simulink model "RC_Model"  (R2023b)
settings: Solver=VariableStepAuto  StartTime=0.0  StopTime=10.0  MaxStep=1e-3  RelTol=1e-3
values from neighbouring files (symbols this model uses):
  C = 1*10^-6    (= 1e-06)    [Script_Rc_model.m]
  R = 1    [Script_Rc_model.m]
settings Model: Creator=gaafa  LastModifiedBy=gaafa

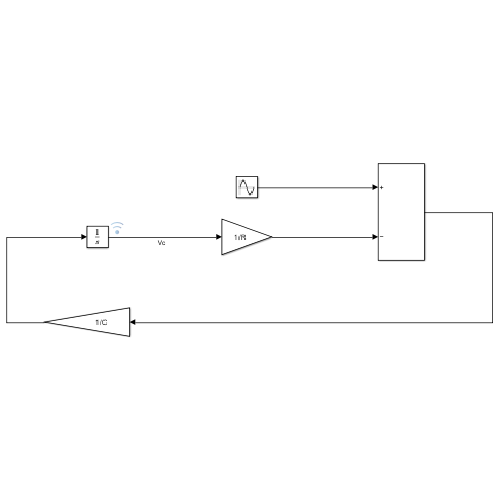
[thumbnail: Simulink's stored preview of the top-level diagram]
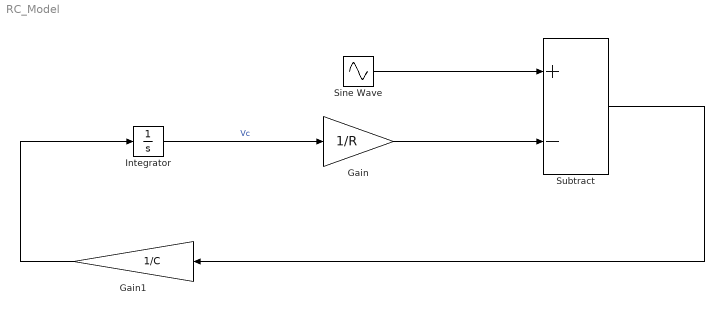
== system RC_Model ==
  Gain : Gain  Gain=1/R
  Gain1 : Gain  Gain=1/C
  Integrator : Integrator
  Sine Wave : Sin  Amplitude=5  Frequency=2*pi  SampleTime=0
  Subtract : Sum  Inputs=+-
  wires:
  Subtract/1 -> Gain1/1
  Integrator/1 -> Gain/1  "Vc"
  Gain/1 -> Subtract/2
  Sine Wave/1 -> Subtract/1
  Gain1/1 -> Integrator/1
